simulink model "Schema"  (R2023a)
settings: Solver=VariableStepAuto  StartTime=0.0  StopTime=15  RelTol=1e-3
undefined symbols (not defined in the file): H1, H2, H3, Kp1, Kp2, Kp3, N1, N2, N3, Td1, Td2, Td3, Ti1, Ti2, Ti3
settings Model: Creator=dandr  LastModifiedBy=dandr

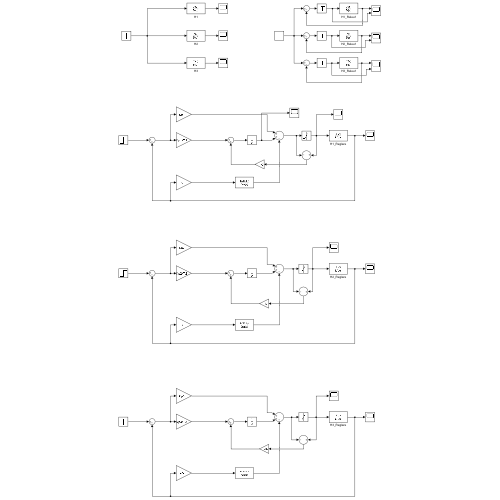
[thumbnail: Simulink's stored preview of the top-level diagram]
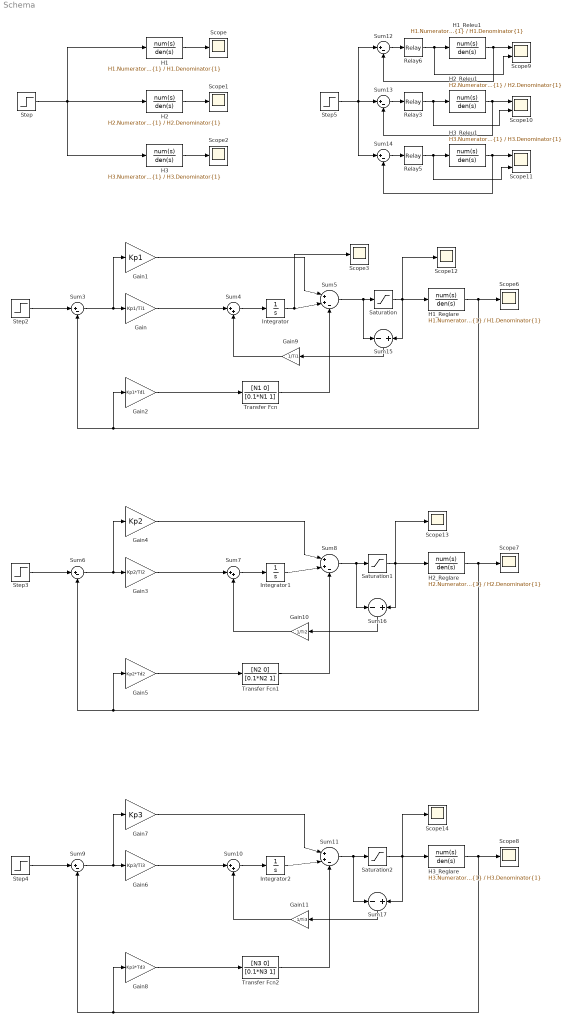
== system Schema ==
  Gain : Gain  Gain=Kp1/Ti1
  Gain1 : Gain  Gain=Kp1
  Gain10 : Gain  Gain=1/Ti2
  Gain11 : Gain  Gain=1/Ti3
  Gain2 : Gain  Gain=Kp1*Td1
  Gain3 : Gain  Gain=Kp2/Ti2
  Gain4 : Gain  Gain=Kp2
  Gain5 : Gain  Gain=Kp2*Td2
  Gain6 : Gain  Gain=Kp3/Ti3
  Gain7 : Gain  Gain=Kp3
  Gain8 : Gain  Gain=Kp3*Td3
  Gain9 : Gain  Gain=1/Ti1
  H1 : TransferFcn  Numerator=H1.Numerator{1}  Denominator=H1.Denominator{1}
  H1_Reglare : TransferFcn  Numerator=H1.Numerator{1}  Denominator=H1.Denominator{1}
  H1_Releu1 : TransferFcn  Numerator=H1.Numerator{1}  Denominator=H1.Denominator{1}
  H2 : TransferFcn  Numerator=H2.Numerator{1}  Denominator=H2.Denominator{1}
  H2_Reglare : TransferFcn  Numerator=H2.Numerator{1}  Denominator=H2.Denominator{1}
  H2_Releu1 : TransferFcn  Numerator=H2.Numerator{1}  Denominator=H2.Denominator{1}
  H3 : TransferFcn  Numerator=H3.Numerator{1}  Denominator=H3.Denominator{1}
  H3_Reglare : TransferFcn  Numerator=H3.Numerator{1}  Denominator=H3.Denominator{1}
  H3_Releu1 : TransferFcn  Numerator=H3.Numerator{1}  Denominator=H3.Denominator{1}
  Integrator : Integrator
  Integrator1 : Integrator
  Integrator2 : Integrator
  Relay3 : Relay  OnSwitchValue=0  OffSwitchValue=0  OnOutputValue=1.5  OffOutputValue=-1.5
  Relay5 : Relay  OnSwitchValue=0  OffSwitchValue=0  OnOutputValue=1.5  OffOutputValue=-1.5  ZeroCross=off
  Relay6 : Relay  OnSwitchValue=0  OffSwitchValue=0  OnOutputValue=5  OffOutputValue=-5
  Saturation : Saturate  UpperLimit=10  LowerLimit=-4
  Saturation1 : Saturate  UpperLimit=1.2  LowerLimit=-0.7
  Saturation2 : Saturate  UpperLimit=2  LowerLimit=-0.2
  Scope{,1..3,6..8,12..14} (10 alike) : Scope
  Scope10 : Scope  NumInputPorts=2
  Scope11 : Scope  NumInputPorts=2
  Scope9 : Scope  NumInputPorts=2
  Step{,2..5} (5 alike) : Step  Time=0  SampleTime=0.01
  Sum10 : Sum  Inputs=|++
  Sum11 : Sum  Inputs=|++-
  Sum{3,6,9,12..14} (6 alike) : Sum  Inputs=|+-
  Sum15 : Sum  Inputs=-|+
  Sum16 : Sum  Inputs=-|+
  Sum17 : Sum  Inputs=-|+
  Sum4 : Sum  Inputs=|++
  Sum5 : Sum  Inputs=|++-
  Sum7 : Sum  Inputs=|++
  Sum8 : Sum  Inputs=|++-
  Transfer Fcn : TransferFcn  Numerator=[N1 0]  Denominator=[0.1*N1 1]
  Transfer Fcn1 : TransferFcn  Numerator=[N2 0]  Denominator=[0.1*N2 1]
  Transfer Fcn2 : TransferFcn  Numerator=[N3 0]  Denominator=[0.1*N3 1]
  wires:
  Step/1 -> H1/1, H3/1, H2/1
  H1/1 -> Scope/1
  H2/1 -> Scope1/1
  H3/1 -> Scope2/1
  Sum3/1 -> Gain1/1, Gain/1
  Step2/1 -> Sum3/1
  Gain/1 -> Sum4/1
  Sum4/1 -> Integrator/1
  Integrator/1 -> Scope3/1, Sum5/2
  Gain1/1 -> Sum5/1
  Sum5/1 -> Sum15/1, Saturation/1
  H1_Reglare/1 -> Sum3/2, Gain2/1, Scope6/1
  Gain2/1 -> Transfer Fcn/1
  Transfer Fcn/1 -> Sum5/3
  Transfer Fcn1/1 -> Sum8/3
  Sum7/1 -> Integrator1/1
  Gain5/1 -> Transfer Fcn1/1
  Gain4/1 -> Sum8/1
  Integrator1/1 -> Sum8/2
  Gain3/1 -> Sum7/1
  H2_Reglare/1 -> Gain5/1, Sum6/2, Scope7/1
  Sum8/1 -> Saturation1/1, Sum16/1
  Step3/1 -> Sum6/1
  Sum6/1 -> Gain4/1, Gain3/1
  H3_Reglare/1 -> Sum9/2, Gain8/1, Scope8/1
  Gain6/1 -> Sum10/1
  Gain7/1 -> Sum11/1
  Sum9/1 -> Gain7/1, Gain6/1
  Sum10/1 -> Integrator2/1
  Step4/1 -> Sum9/1
  Gain8/1 -> Transfer Fcn2/1
  Integrator2/1 -> Sum11/2
  Transfer Fcn2/1 -> Sum11/3
  H1_Releu1/1 -> Sum12/2, Scope9/1
  H3_Releu1/1 -> Sum14/2, Scope11/1
  Sum14/1 -> Relay5/1
  Sum13/1 -> Relay3/1
  Relay6/1 -> Scope9/2, H1_Releu1/1
  Step5/1 -> Sum14/1, Sum13/1, Sum12/1
  Sum12/1 -> Relay6/1
  Relay3/1 -> Scope10/2, H2_Releu1/1
  Relay5/1 -> Scope11/2, H3_Releu1/1
  H2_Releu1/1 -> Sum13/2, Scope10/1
  Saturation/1 -> Scope12/1, Sum15/2, H1_Reglare/1
  Saturation1/1 -> Scope13/1, Sum16/2, H2_Reglare/1
  Sum11/1 -> Saturation2/1, Sum17/1
  Sum15/1 -> Gain9/1
  Sum16/1 -> Gain10/1
  Gain10/1 -> Sum7/2
  Sum17/1 -> Gain11/1
  Gain11/1 -> Sum10/2
  Saturation2/1 -> Sum17/2, H3_Reglare/1, Scope14/1
  Gain9/1 -> Sum4/2
